simulink model "SEPIC_V1_SIMU"  (R2017b)
settings: Solver=ode23t  StartTime=0.0  StopTime=0.2  MaxStep=100e-9  RelTol=100e-9
values from neighbouring files (symbols this model uses):
  C = 56*10^-6    (= 5.6e-05)    [CODIGO_MATLAB_PLANTA_ESTABILIDAD_CONTROLADOR.m]    (also in PLANT STABILITY.m; PLANT_STABILITY.m)
  CIN = 56*10^-6    (= 5.6e-05)    [CODIGO_MATLAB_PLANTA_ESTABILIDAD_CONTROLADOR.m]    (also in PLANT STABILITY.m; PLANT_STABILITY.m)
  CX = 56*10^-6    (= 5.6e-05)    [CODIGO_MATLAB_PLANTA_ESTABILIDAD_CONTROLADOR.m]    (also in PLANT STABILITY.m; PLANT_STABILITY.m)
  ESR = 0.029    [CODIGO_MATLAB_PLANTA_ESTABILIDAD_CONTROLADOR.m]    (also in PLANT STABILITY.m; PLANT_STABILITY.m)
  L = 220*10^-6    (= 0.00022)    [CODIGO_MATLAB_PLANTA_ESTABILIDAD_CONTROLADOR.m]    (also in PLANT STABILITY.m; PLANT_STABILITY.m)
  RSH = 0.1    [CODIGO_MATLAB_PLANTA_ESTABILIDAD_CONTROLADOR.m]    (also in PLANT STABILITY.m; PLANT_STABILITY.m)
  VO = 14.7    [CODIGO_MATLAB_PLANTA_ESTABILIDAD_CONTROLADOR.m]    (also in PLANT STABILITY.m; PLANT_STABILITY.m)
undefined symbols (not defined in the file or in its folder): Acid, Lead
libraries: powerlib x28, electricdrivelib x1, re_lib x1
settings Model: Creator=TG1748  LastModifiedBy=arman
settings SolverCC: ZeroCrossAlgorithm=Adaptive
settings DebuggingCC: UnconnectedInputMsg=none  UnconnectedOutputMsg=none  UnconnectedLineMsg=none
settings ConfigComp: PLC_TargetIDE=codesys23  PLC_GenerateReport=off  PLC_LaunchReport=off

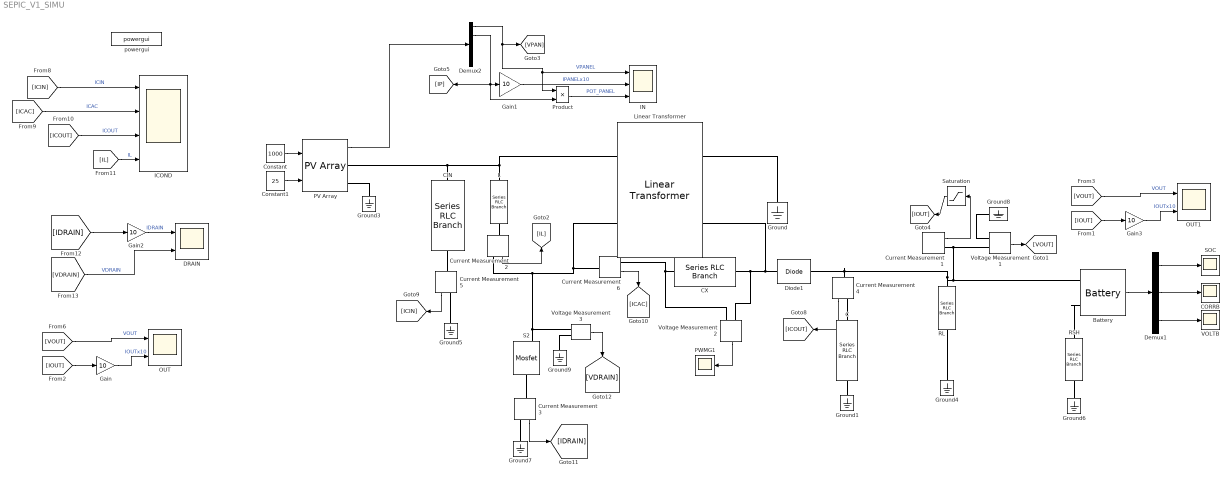
== system SEPIC_V1_SIMU ==
  Battery : electricdrivelib/Extra Sources/Battery  BatType=Lead-Acid  ShowTempParam=off  ThermalPreset=no  ShowAgeParam=off  NomV=12  NomQ=7.2  SOC=50  Batt_Tr=30  PresetModel=off  MaxQ=7.5  MinV=9  FullV=14.7  Dis_rate=0.375  R=0.024  Normal_OP=6  expZone="[12.8        0.024]"  current=[0.375 0.746 1.32]  Units=Time  Tci=20  NomT=20  T2=-30  MaxQ2=4.8  FullV2=7.1  Normal_OP2=5.655  expZone2="[6.58           1]"  Rca=0.6  ti=2000  Dp=0  Neq0=0  Tsim=1e6  Ta1=25  Qeol=5.4*0.9  Reol=0.013333*1.2  Char_age=[2.3478, 3]  Dis_age=[2.3478, 10]  N1=1500  N2=10500  N3=1000  N4=1400  Ta2=45  N5=950
  C : powerlib/Elements/Series RLC Branch  LConnTagsString=__new0  RConnTagsString=__new0  BranchType=RC  Resistance=ESR  Inductance=1e-3  SetiL0=off  InitialCurrent=0  Capacitance=C  Setx0=off  InitialVoltage=0  Measurements=None
  CIN : powerlib/Elements/Series RLC Branch  LConnTagsString=__new0  RConnTagsString=__new0  BranchType=RC  Resistance=ESR  Inductance=1e-3  SetiL0=off  InitialCurrent=0  Capacitance=CIN  Setx0=off  InitialVoltage=0  Measurements=None
  CORRB : Scope
  CX : powerlib/Elements/Series RLC Branch  LConnTagsString=__new0  RConnTagsString=__new0  BranchType=RC  Resistance=ESR  Inductance=1e-3  SetiL0=off  InitialCurrent=0  Capacitance=CX  Setx0=off  InitialVoltage=0  Measurements=None
  Constant : Constant  Value=1000
  Constant1 : Constant  Value=25
  Current Measurement{1..6} (6 alike) : powerlib/Measurements/Current Measurement  PhasorSimulation=off  OutputType=Complex  PSBequivalent=0
  DRAIN : Scope  NumInputPorts=2
  Demux1 : Demux  Outputs=3
  Demux2 : Demux  Outputs=5
  Diode1 : powerlib/Power Electronics/Diode  Ron=0.001  Lon=0  Vf=VD  IC=0  UseSnubber=off  Rs=inf  Cs=250e-9  Measurements=off
  Gain{,1..3} (4 alike) : Gain  Gain=10
  Ground{,1,3..9} (9 alike) : powerlib/Elements/Ground  LConnTagsString=a
  ICOND : Scope  NumInputPorts=4
  IN : Scope  NumInputPorts=3
  L : powerlib/Elements/Series RLC Branch  LConnTagsString=__new0  RConnTagsString=__new0  BranchType=L  Resistance=1  Inductance=L  SetiL0=off  InitialCurrent=0  Capacitance=1e-6  Setx0=off  InitialVoltage=0  Measurements=None
  Linear Transformer : powerlib/Elements/Linear Transformer  UNITS=SI  NominalPower=[ 22 100000 ]  winding1=[1 0 0]  winding2=[1 0 0]  ThreeWindings=off  winding3=[3.15e+05 0.7938 0.084225]  RmLm=[1e6 inf]  Measurements=None  DataType=on
  OUT : Scope  NumInputPorts=2
  OUT1 : Scope  NumInputPorts=2
  PV Array : re_lib/Solar/PV Array  Npar=1  Nser=1  PlotType=array @ 25 deg.C & specified irradiances  S_vec="[ 1000  500  100 ]"  Temp_C_vec="[ 45 25  ]"  ModuleName=User-defined  PlotWhenSelected=off  Pm=19.95  Ncell=36  Voc=21.6  Isc=1.23  Vm=17.5  Im=1.14  beta_Voc_pc=-0.333  alpha_Isc_pc=0.05  beta_Voc=-0.071928  alpha_Isc=0.000615  IL=1.239  I0=1.5415e-11  nI=0.93147  Rsh=462.7836  Rs=1.3323  BAL=on  Tc=1e-6  Tfilter=5e-5
  PWMG1 : Scope
  Product : Product
  RL : powerlib/Elements/Series RLC Branch  LConnTagsString=__new0  RConnTagsString=__new0  BranchType=R  Resistance=VO  Inductance=1e-3  SetiL0=off  InitialCurrent=0  Capacitance=1e-6  Setx0=off  InitialVoltage=0  Measurements=None
  RSH : powerlib/Elements/Series RLC Branch  LConnTagsString=__new0  RConnTagsString=__new0  BranchType=R  Resistance=RSH  Inductance=1e-3  SetiL0=off  InitialCurrent=0  Capacitance=1e-6  Setx0=off  InitialVoltage=0  Measurements=None
  S2 : powerlib/Power Electronics/Mosfet  Ron=0.007  Lon=0  Rd=0.0062  Vfd=1.3  IC=0  Rs=1e5  Cs=inf  Measurements=off
  SOC : Scope
  Saturation : Saturate  UpperLimit=1.5  LowerLimit=0
  VOLTB : Scope
  Voltage Measurement1 : powerlib/Measurements/Voltage Measurement  PhasorSimulation=off  OutputType=Complex  PSBequivalent=0
  Voltage Measurement2 : powerlib/Measurements/Voltage Measurement  PhasorSimulation=off  OutputType=Complex  PSBequivalent=0
  Voltage Measurement3 : powerlib/Measurements/Voltage Measurement  PhasorSimulation=off  OutputType=Complex  PSBequivalent=0
  powergui : powerlib/powergui  SimulationMode=Continuous  SampleTime=50e-6  frequency=60  Iterations=50  frequencyindice=0  Pbase=100e6  ErrMax=1e-4  UnitsV=kV  UnitsW=MW  buscounter=0  FunctionMessages=off  echomessages=off  EnableUseOfTLC=off  CurrentSourceSwitches=off  DisableSnubberDevices=off  DisableRonSwitches=off  DisableVfSwitches=off  DisplayEquations=off  SolverType=Tustin/Backward Euler (TBE)  Interpol=off  ExternalGateDelay=off  methode=off  Ts=100  x0status=blocks  SPID=on  SwTol=0  HookPort=off  RestoreLinks=warning  ResistiveCurrentMeasurement=off  Frange=[0:2:500]  Ylog=off  Xlog=on  ShowGrid=off  save=off  variable=ZData  structure=0  ZoomFFT=on  StartTime=0.0  cycles=1  DisplayStyle=1  fundamental=60  FreqAxis=off  MaxFrequency=1000  frequencyindicesteady=1  RmsSteady=1  display=off
  wires:
  Constant/1 -> PV Array/1
  Constant1/1 -> PV Array/2
  PV Array/1 -> Demux2/1
  Current Measurement2/1 -> [IL]
  [VOUT] -> OUT/1  "VOUT"
  [IOUT] -> Gain/1
  Gain/1 -> OUT/2  "IOUTx10"
  Demux2/1 -> [VPAN], IN/1, Product/1  "VPANEL"
  Product/1 -> IN/3  "POT_PANEL"
  Current Measurement4/1 -> [ICOUT]
  Current Measurement5/1 -> [ICIN]
  Current Measurement6/1 -> [ICAC]
  [ICAC] -> ICOND/2  "ICAC"
  [ICOUT] -> ICOND/3  "ICOUT"
  [IL] -> ICOND/4  "IL"
  Voltage Measurement2/1 -> PWMG1/1
  Gain2/1 -> DRAIN/1  "IDRAIN"
  [IDRAIN] -> Gain2/1
  Voltage Measurement3/1 -> [VDRAIN]
  Current Measurement3/1 -> [IDRAIN]
  [ICIN] -> ICOND/1  "ICIN"
  Demux2/2 -> [IP], Product/2, Gain1/1
  Gain1/1 -> IN/2  "IPANELx10"
  [VDRAIN] -> DRAIN/2  "VDRAIN"
  Demux1/2 -> CORRB/1
  Demux1/3 -> VOLTB/1
  Battery/1 -> Demux1/1
  Demux1/1 -> SOC/1
  [VOUT] -> OUT1/1  "VOUT"
  Saturation/1 -> [IOUT]
  [IOUT] -> Gain3/1
  Gain3/1 -> OUT1/2  "IOUTx10"
  Current Measurement1/1 -> Saturation/1
  Voltage Measurement1/1 -> [VOUT]
  connections:
  Voltage Measurement1/LConn1 -- RL/LConn1 -- Current Measurement4/LConn1 -- Diode1/RConn1 -- Battery/LConn1 -- Current Measurement1/RConn1
  Diode1/LConn1 -- Voltage Measurement2/LConn2 -- CX/RConn1 -- Linear Transformer/RConn1
  CIN/LConn1 -- PV Array/RConn1 -- Linear Transformer/LConn2 -- L/LConn1
  Ground/LConn1 -- Linear Transformer/RConn2
  PV Array/RConn2 -- Ground3/LConn1
  L/RConn1 -- Current Measurement2/LConn1
  Linear Transformer/LConn1 -- Current Measurement2/RConn1 -- Voltage Measurement3/LConn1 -- S2/LConn1 -- Current Measurement6/LConn1
  Current Measurement6/RConn1 -- Voltage Measurement2/LConn1 -- CX/LConn1
  Ground5/LConn1 -- Current Measurement5/RConn1
  CIN/RConn1 -- Current Measurement5/LConn1
  Current Measurement4/RConn1 -- C/LConn1
  Ground1/LConn1 -- C/RConn1
  Current Measurement3/LConn1 -- S2/RConn1
  Ground7/LConn1 -- Current Measurement3/RConn1
  Ground9/LConn1 -- Voltage Measurement3/LConn2
  Battery/LConn2 -- RSH/LConn1
  RSH/RConn1 -- Ground6/LConn1
  RL/RConn1 -- Ground4/LConn1
  Ground8/LConn1 -- Voltage Measurement1/LConn2
